simulink model "MobileRobot"  (R2024b)
settings: Solver=VariableStepAuto  StartTime=0.0  StopTime=40  RelTol=1e-3
model workspace (MAT data in the model file):
  PasDeTemps = 0.01
undefined symbols (not defined in the file or in its folder): magnitude, TimeStep
libraries: sharedTrackingLibrary x1, simulink x1, dspsigops x1, robotmobilelib x1
settings Model: Creator=p22524  LastModifiedBy=p22524

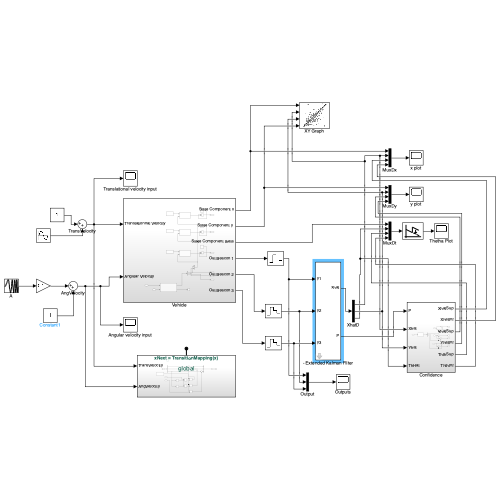
[thumbnail: Simulink's stored preview of the top-level diagram]
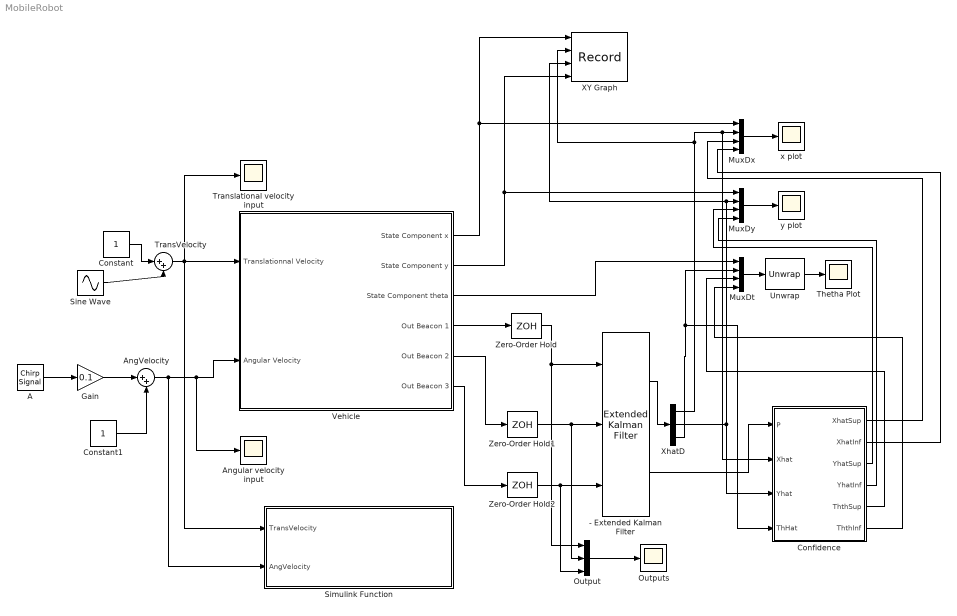
== system MobileRobot ==
  - Extended Kalman Filter : sharedTrackingLibrary/Extended Kalman Filter  StateTransitionFcn=TransitionMapping  HasStateTransitionJacobianFcn=off  HasAdditiveProcessNoise=Additive  ProcessNoise=0.01*diag([1 1 1])  HasTimeVaryingProcessNoise=off  HasStateTransitionFcnExtraArgument=0  InitialState=[10,10,1]  InitialStateCovariance=1*diag([1,1,1])  MeasurementFcn1=DistanceBalise1  HasMeasurementJacobianFcn1=off  HasMeasurementEnablePort1=off  HasAdditiveMeasurementNoise1=Additive  MeasurementNoise1=0.0025  HasTimeVaryingMeasurementNoise1=off  HasMeasurementFcnExtraArgument1=0  HasMeasurementWrapping1=off  MeasurementFcn2=DistanceBalise2  HasMeasurementJacobianFcn2=off  HasMeasurementEnablePort2=off  HasAdditiveMeasurementNoise2=Additive  MeasurementNoise2=0.0025  HasTimeVaryingMeasurementNoise2=off  HasMeasurementFcnExtraArgument2=0  HasMeasurementWrapping2=off  MeasurementFcn3=DistanceBalise3  HasMeasurementJacobianFcn3=off  HasMeasurementEnablePort3=off  HasAdditiveMeasurementNoise3=Additive  MeasurementNoise3=0.0025  HasTimeVaryingMeasurementNoise3=off  HasMeasurementFcnExtraArgument3=0  HasMeasurementWrapping3=off  MeasurementFcn4=myMeasurementFcn  HasMeasurementJacobianFcn4=off  HasMeasurementEnablePort4=off  HasAdditiveMeasurementNoise4=Additive  MeasurementNoise4=1  HasTimeVaryingMeasurementNoise4=off  HasMeasurementFcnExtraArgument4=0  HasMeasurementWrapping4=off  MeasurementFcn5=myMeasurementFcn  HasMeasurementJacobianFcn5=off  HasMeasurementEnablePort5=off  HasAdditiveMeasurementNoise5=Additive  MeasurementNoise5=1  HasTimeVaryingMeasurementNoise5=off  HasMeasurementFcnExtraArgument5=0  HasMeasurementWrapping5=off  EnableMultirate=on  StateTransitionFcnSampleTime=TimeStep  MeasurementFcn1SampleTime=0.02  MeasurementFcn2SampleTime=0.02  MeasurementFcn3SampleTime=0.02  MeasurementFcn4SampleTime=1  MeasurementFcn5SampleTime=1  UseCurrentEstimator=on  OutputStateCovariance=on  DataType=double  SampleTime=1  NumberOfMeasurements=3
  "A " : simulink/Sources/Chirp Signal  f1=0.1  T=10  f2=1
  AngVelocity : Sum  Inputs=|++
  Angular velocity input : Scope
  Confidence : Subsystem
  Constant : Constant
  Constant1 : Constant
  Gain : Gain  Gain=0.1
  MuxDt : Mux
  MuxDx : Mux
  MuxDy : Mux
  Output : Mux  Inputs=3
  Outputs : Scope
  Simulink Function : Subsystem  TreatAsAtomicUnit=on
  Sine Wave : Sin  Amplitude=0.5  SampleTime=0
  Thetha Plot : Scope
  TransVelocity : Sum  Inputs=|++
  Translational velocity input : Scope
  Unwrap : dspsigops/Unwrap  tol=pi  InputProcessing=Columns as channels (frame based)  running=off
  Vehicle : Subsystem
  XY Graph : Record  FileSettingsInternal="{\"entries\":[{\"content\":{\"excelSettings\":{\"content\":{},\"type\":\"Streamout.ExcelSettings\"}},\"type\":\"Streamout.FileSettingStorage\",\"uuid\":\"\"}],\"packageUris\":[\"http:\\/\\/schema.mathworks.com\\/mf0\\/streamout_blocks\\/R2020a\"],\"version\":\"1.0\"}"  Layout=[1 1]  SignalsInternal="{\"entries\":[{\"content\":{\"signals\":[{\"content\":{\"blockPath\":[],\"dimensions\":[1],\"domain\":\"\",\"lineColor\":\"#a2142f\",\"plots\":[ 1 ],\"port\":1,\"sid\":[\"\"],\"signalID\":1,\"signalName\":\"Vehicle:1\"},\"type\":\"RecordBlkView.Signal\",\"uuid\":\"\"},{\"content\":{\"blockPath\":[],\"dimensions\":[1],\"domain\":\"\",\"lineColor\":\"#139fff\",\"plots\":[ 1 ],\"port\":2,\"sid\":[\"\"],\"signalID\":2,\"signalName\":\"XhatD:1\"},\"type\":\"RecordBlkView.Signal\",\"uuid\":\"\"},{\"content\":{\"blockPath\":[],\"dimensions\":[1],\"domain\":\"\",\"lineColor\":\"#77ac30\",\"lineWidth\":2,\"plots\":[ 1 ],\"port\":3,\"sid\":[\"\"],\"signalID\":3,\"signalName\":\"XhatD:2\"},\"type\":\"RecordBlkView.Signal\",\"uuid\":\"\"},{\"content\":{\"blockPath\":[],\"dimensions\":[1],\"domain\":\"\",\"lineColor\":\"#4dbeee\",\"lineWidth\":2,\"plots\":[ 1 ],\"port\":4,\"sid\":[\"\"],\"signalID\":4,\"signalName\":\"Vehicle:2\"},\"type\":\"RecordBlkView.Signal\",\"uuid\":\"\"}]},\"type\":\"RecordBlkView.InputSignals\",\"uuid\":\"\"}],\"packageUris\":[\"http:\\/\\/schema.mathworks.com\\/mf0\\/streamout_blocks\\/R2020a\"],\"version\":\"1.0\"}"  VisualizationBindings="{\"xyplotplugin\":{\"info\":[{\"series\":[{\"bindingParametersList\":[{\"parameter\":\"X-Axis\",\"signalID\":1,\"signalName\":\"Vehicle:1\"},{\"parameter\":\"Y-Axis\",\"signalID\":4,\"signalName\":\"Vehicle:2\"},{\"parameter\":\"X-Axis\",\"signalID\":1,\"signalName\":\"Vehicle:1\"},{\"parameter\":\"Y-Axis\",\"signalID\":4,\"signalName\":\"Vehicle:2\"}],\"seriesID\":0},{\"bindingParametersList\":[{\"parameter\":\"X-Axis\",\"signalID\":2,\"signalName\":\"XhatD:1\"},{\"parameter\":\"Y-Axis\",\"signalID\":3,\"signalName\":\"XhatD:2\"},{\"parameter\":\"X-Axis\",\"signalID\":2,\"signalName\":\"XhatD:1\"},{\"parameter\":\"Y-Axis\",\"signalID\":3,\"signalName\":\"XhatD:2\"}],\"seriesID\":1}],\"subplotID\":1}]}}"  CompatibilityTag=XY
  XhatD : Demux  Outputs=3
  Zero-Order Hold : ZeroOrderHold  SampleTime=0.02
  Zero-Order Hold1 : ZeroOrderHold  SampleTime=0.02
  Zero-Order Hold2 : ZeroOrderHold  SampleTime=0.02
  x plot : Scope
  y plot : Scope
  wires:
  Vehicle/2("State Component y ") -> MuxDy/1, XY Graph/4
  Vehicle/3(State Component theta) -> MuxDt/1
  MuxDx/1 -> x plot/1
  Vehicle/1(State Component x) -> XY Graph/1, MuxDx/1
  Zero-Order Hold/1 -> Output/1, - Extended Kalman Filter/1
  Zero-Order Hold2/1 -> - Extended Kalman Filter/3, Output/3
  Zero-Order Hold1/1 -> - Extended Kalman Filter/2, Output/2
  Vehicle/5(Out Beacon 2) -> Zero-Order Hold1/1
  Constant/1 -> TransVelocity/1
  TransVelocity/1 -> Vehicle/1(Translationnal Velocity), Translational velocity input/1, Simulink Function/1(TransVelocity)
  - Extended Kalman Filter/1 -> XhatD/1
  XhatD/1 -> XY Graph/2, Confidence/2(Xhat), MuxDx/2
  MuxDy/1 -> y plot/1
  XhatD/2 -> MuxDy/2, XY Graph/3, Confidence/3(Yhat)
  XhatD/3 -> Confidence/4(ThHat), MuxDt/2
  MuxDt/1 -> Unwrap/1
  Vehicle/4(Out Beacon 1) -> Zero-Order Hold/1
  Vehicle/6(Out Beacon 3) -> Zero-Order Hold2/1
  Output/1 -> Outputs/1
  - Extended Kalman Filter/2 -> Confidence/1(P)
  Confidence/1(XhatSup) -> MuxDx/3
  Confidence/2(XhatInf) -> MuxDx/4
  Confidence/3(YhatSup) -> MuxDy/3
  Confidence/4(YhatInf) -> MuxDy/4
  Confidence/5(ThthSup) -> MuxDt/3
  Confidence/6(ThthInf) -> MuxDt/4
  Sine Wave/1 -> TransVelocity/2
  AngVelocity/1 -> Simulink Function/2(AngVelocity), Angular velocity input/1, Vehicle/2(Angular Velocity)
  Constant1/1 -> AngVelocity/2
  Gain/1 -> AngVelocity/1
  "A "/1 -> Gain/1
  Unwrap/1 -> Thetha Plot/1

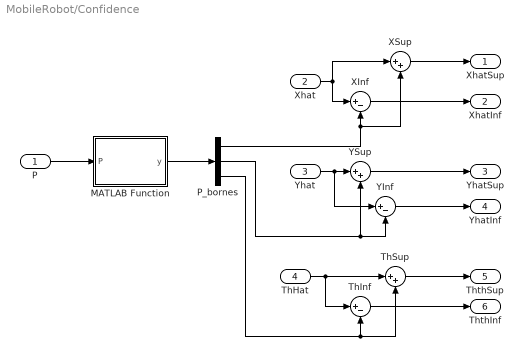
== system MobileRobot/Confidence ==
  P : Inport
  Xhat : Inport  Port=2
  Yhat : Inport  Port=3
  ThHat : Inport  Port=4
  MATLAB Function : MATLAB Function  TreatAsAtomicUnit=on
  P_bornes : Demux  Outputs=3
  ThInf : Sum  Inputs=|+-
  ThSup : Sum  Inputs=|++
  XInf : Sum  Inputs=|+-
  XSup : Sum  Inputs=|++
  YInf : Sum  Inputs=|+-
  YSup : Sum  Inputs=|++
  XhatSup : Outport
  XhatInf : Outport  Port=2
  YhatSup : Outport  Port=3
  YhatInf : Outport  Port=4
  ThthSup : Outport  Port=5
  ThthInf : Outport  Port=6
  wires:
  P/1 -> MATLAB Function/1(P)
  XInf/1 -> XhatInf/1
  YInf/1 -> YhatInf/1
  ThInf/1 -> ThthInf/1
  P_bornes/2 -> YInf/2, YSup/2
  XSup/1 -> XhatSup/1
  Xhat/1 -> XSup/1, XInf/1
  MATLAB Function/1(y) -> P_bornes/1
  Yhat/1 -> YInf/1, YSup/1
  ThSup/1 -> ThthSup/1
  P_bornes/3 -> ThSup/2, ThInf/2
  ThHat/1 -> ThInf/1, ThSup/1
  YSup/1 -> YhatSup/1
  P_bornes/1 -> XSup/2, XInf/2

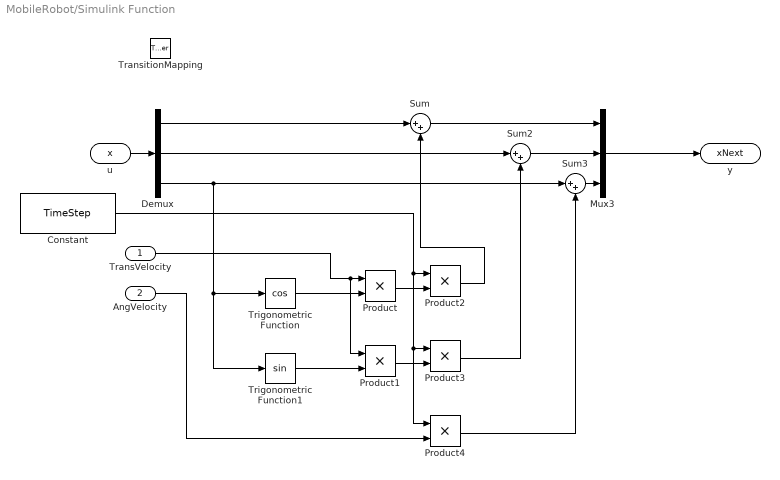
== system MobileRobot/Simulink Function ==
  TransVelocity : Inport
  AngVelocity : Inport  Port=2
  TransitionMapping : TriggerPort  TriggerType=function-call  IsSimulinkFunction=on  FunctionName=TransitionMapping  VariantControl=(inherit)
  Constant : Constant  Value=TimeStep
  Demux : Demux  Outputs=3
  Mux3 : Mux  Inputs=3
  Product{,1..4} (5 alike) : Product
  Sum : Sum  Inputs=|++
  Sum2 : Sum  Inputs=|++
  Sum3 : Sum  Inputs=|++
  Trigonometric Function : Trigonometry  Operator=cos
  Trigonometric Function1 : Trigonometry
  u : ArgIn  DisableCoverage=on  PortDimensions=3  ArgumentName=x
  y : ArgOut  DisableCoverage=on  PortDimensions=3  ArgumentName=xNext
  wires:
  u/1 -> Demux/1
  Trigonometric Function/1 -> Product/2
  TransVelocity/1 -> Product1/1, Product/1
  Trigonometric Function1/1 -> Product1/2
  Demux/1 -> Sum/1
  Sum/1 -> Mux3/1
  Demux/2 -> Sum2/1
  Product/1 -> Product2/2
  Product1/1 -> Product3/2
  Constant/1 -> Product4/1, Product3/1, Product2/1
  Product2/1 -> Sum/2
  Product3/1 -> Sum2/2
  Sum2/1 -> Mux3/2
  Demux/3 -> Trigonometric Function1/1, Trigonometric Function/1, Sum3/1
  Sum3/1 -> Mux3/3
  AngVelocity/1 -> Product4/2
  Product4/1 -> Sum3/2
  Mux3/1 -> y/1

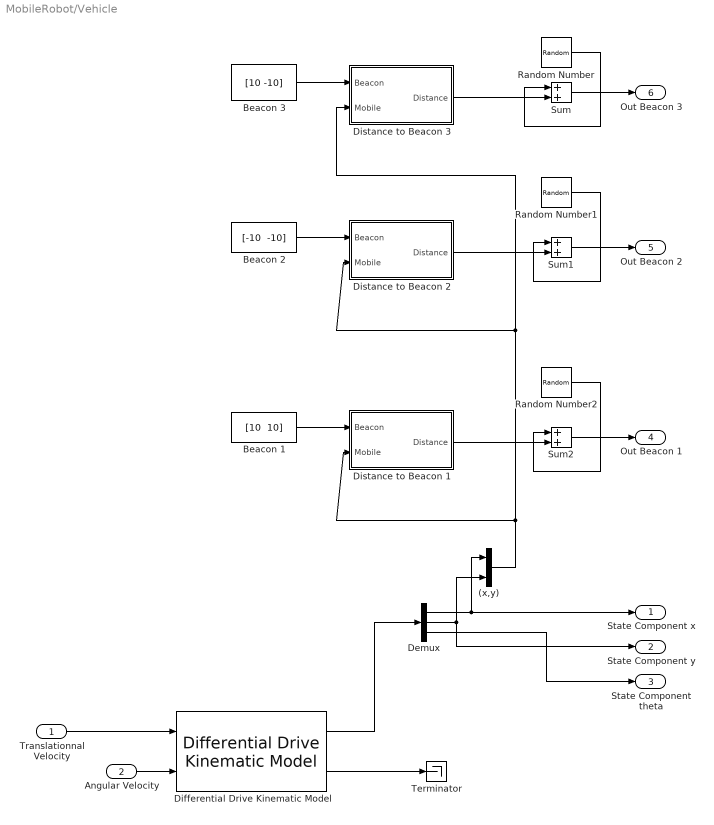
== system MobileRobot/Vehicle ==
  Translationnal Velocity : Inport
  Angular Velocity : Inport  Port=2
  (x,y) : Mux  Inputs=2
  Beacon 1 : Constant  Value="[10  10]"
  Beacon 2 : Constant  Value="[-10  -10]"
  Beacon 3 : Constant  Value=[10 -10]
  Demux : Demux  Outputs=3
  Differential Drive Kinematic Model : robotmobilelib/Differential Drive Kinematic Model  VehicleInputs=Vehicle Speed & Heading Angular Velocity  WheelRadius=0.05  WheelSpeedRange=[-inf inf]  TrackWidth=0.2  InitialState=[-5; 5; 0]  SimulateUsing=Code generation
  Distance to Beacon 1 : Subsystem
  Distance to Beacon 2 : Subsystem
  Distance to Beacon 3 : Subsystem
  Random Number : RandomNumber  Variance=0.0025  SampleTime=PasDeTemps
  Random Number1 : RandomNumber  Variance=0.0025  SampleTime=PasDeTemps
  Random Number2 : RandomNumber  Variance=0.0025  SampleTime=PasDeTemps
  Sum : Sum
  Sum1 : Sum
  Sum2 : Sum
  Terminator : Terminator
  State Component x : Outport
  "State Component y " : Outport  Port=2
  State Component theta : Outport  Port=3
  Out Beacon 1 : Outport  Port=4
  Out Beacon 2 : Outport  Port=5
  Out Beacon 3 : Outport  Port=6
  wires:
  Distance to Beacon 1/1(Distance) -> Sum2/2
  Random Number1/1 -> Sum1/1
  Sum1/1 -> Out Beacon 2/1
  Beacon 1/1 -> Distance to Beacon 1/1(Beacon)
  Differential Drive Kinematic Model/2 -> Terminator/1
  Distance to Beacon 3/1(Distance) -> Sum/2
  Sum2/1 -> Out Beacon 1/1
  Sum/1 -> Out Beacon 3/1
  Random Number2/1 -> Sum2/1
  Differential Drive Kinematic Model/1 -> Demux/1
  Demux/1 -> State Component x/1, (x,y)/1
  Angular Velocity/1 -> Differential Drive Kinematic Model/2
  Distance to Beacon 2/1(Distance) -> Sum1/2
  Demux/2 -> "State Component y "/1, (x,y)/2
  Demux/3 -> State Component theta/1
  Random Number/1 -> Sum/1
  (x,y)/1 -> Distance to Beacon 3/2(Mobile), Distance to Beacon 2/2(Mobile), Distance to Beacon 1/2(Mobile)
  Translationnal Velocity/1 -> Differential Drive Kinematic Model/1
  Beacon 3/1 -> Distance to Beacon 3/1(Beacon)
  Beacon 2/1 -> Distance to Beacon 2/1(Beacon)

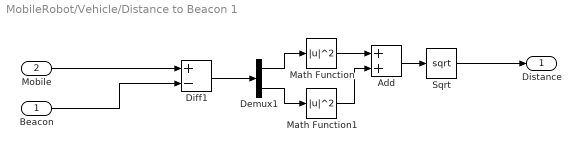
== system MobileRobot/Vehicle/Distance to Beacon 1 ==
  Beacon : Inport
  Mobile : Inport  Port=2
  Add : Sum
  Demux1 : Demux  Outputs=2
  Diff1 : Sum  Inputs=+-
  Math Function : Math  Operator=magnitude^2
  Math Function1 : Math  Operator=magnitude^2
  Sqrt : Sqrt
  Distance : Outport
  wires:
  Beacon/1 -> Diff1/2
  Sqrt/1 -> Distance/1
  Demux1/1 -> Math Function/1
  Add/1 -> Sqrt/1
  Math Function/1 -> Add/1
  Math Function1/1 -> Add/2
  Diff1/1 -> Demux1/1
  Mobile/1 -> Diff1/1
  Demux1/2 -> Math Function1/1

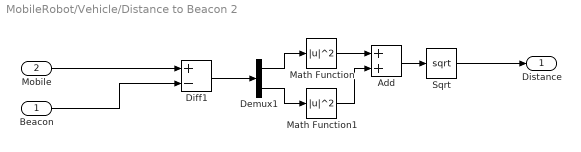
== system MobileRobot/Vehicle/Distance to Beacon 2 ==
  Beacon : Inport
  Mobile : Inport  Port=2
  Add : Sum
  Demux1 : Demux  Outputs=2
  Diff1 : Sum  Inputs=+-
  Math Function : Math  Operator=magnitude^2
  Math Function1 : Math  Operator=magnitude^2
  Sqrt : Sqrt
  Distance : Outport
  wires:
  Beacon/1 -> Diff1/2
  Sqrt/1 -> Distance/1
  Demux1/1 -> Math Function/1
  Add/1 -> Sqrt/1
  Math Function/1 -> Add/1
  Math Function1/1 -> Add/2
  Diff1/1 -> Demux1/1
  Mobile/1 -> Diff1/1
  Demux1/2 -> Math Function1/1

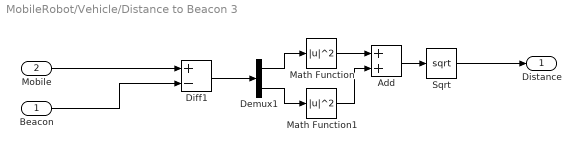
== system MobileRobot/Vehicle/Distance to Beacon 3 ==
  Beacon : Inport
  Mobile : Inport  Port=2
  Add : Sum
  Demux1 : Demux  Outputs=2
  Diff1 : Sum  Inputs=+-
  Math Function : Math  Operator=magnitude^2
  Math Function1 : Math  Operator=magnitude^2
  Sqrt : Sqrt
  Distance : Outport
  wires:
  Beacon/1 -> Diff1/2
  Sqrt/1 -> Distance/1
  Demux1/1 -> Math Function/1
  Add/1 -> Sqrt/1
  Math Function/1 -> Add/1
  Math Function1/1 -> Add/2
  Diff1/1 -> Demux1/1
  Mobile/1 -> Diff1/1
  Demux1/2 -> Math Function1/1

== matlab function MobileRobot/Confidence/MATLAB Function ==
  data: P input; y output
function y = fcn_bornes(P)
% calcul la boite englobante l'ellipsoide matrice de forme P
eta = 0.95;
a = sqrt(-2*log(1-eta ));
QQ = sqrtm(a*P);
y = zeros(3,1);
for i=1:3
    y(i) = norm(QQ(i,:),2);
end
